simulink model "esp32_digital_output_demo"  (R2022a)
settings: Solver=FixedStepDiscrete  StartTime=0.0  StopTime=inf  RelTol=1e-3  EnableMultiTasking=on
undefined symbols (not defined in the file): ESP, IDF
libraries: simulink x9, esp32_io_lib x1, esp32_device_config_lib x1
settings Model: Creator=rnd1  LastModifiedBy=62-603
settings SolverCC: AlgebraicLoopSolver=TrustRegion  PositivePriorityOrder=on  AutoInsertRateTranBlk=on
settings DataIOCC: ReturnWorkspaceOutputs=off
settings OptimizationCC: DefaultParameterBehavior=Inlined  EnhancedBackFolding=on  PassReuseOutputArgsAs=Individual arguments  OptimizeBlockOrder=speed  DifferentSizesBufferReuse=on  OptimizationCustomize=off  EfficientTunableParamExpr=on
settings DebuggingCC: ParameterTunabilityLossMsg=error  UnconnectedInputMsg=warning  UnconnectedOutputMsg=warning  UnconnectedLineMsg=warning  SFMachineParentedDataDiag=warning  ArithmeticOperatorsInVariantConditions=warning
settings HardwareCC: ProdBitPerPointer=32  ProdBitPerSizeT=32  ProdBitPerPtrDiffT=32  ProdLargestAtomicFloat=None  ProdIntDivRoundTo=Undefined  ProdEndianess=Unspecified  ProdWordSize=32  ProdHWDeviceType=Cadence Design Systems (Tensilica)->Xtensa® single-/dual-core 32-bit LX6 microprocessor
settings SFSimCC: MATLABDynamicMemAlloc=off  CustomCodeUndefinedFunction=UseInterfaceOnly
settings RTWCC: Description=Waijung 2 ESP32 target  SystemTargetFile=esp32.tlc  GenCodeOnly=on  MakeCommand=make_rtw TMF=1  GenerateMakefile=off  TemplateMakefile=ert_default_tmf  GenerateReport=on  RetainRTWFile=on  IncludeHyperlinkInReport=on  LaunchReport=on  GenerateTraceInfo=on  GenerateTraceReport=on  GenerateTraceReportSl=on  GenerateTraceReportSf=on  GenerateTraceReportEml=on
settings CodeAppCC: ForceParamTrailComments=on  IgnoreCustomStorageClasses=off  OperatorAnnotations=on  SimulinkDataObjDesc=on  SFDataObjDesc=on  InsertBlockDesc=on
settings ERTTargetCC: TargetLangStandard=C99 (ISO)  UseToolchainInfoCompliant=off  InlinedParameterPlacement=NonHierarchical  ERTSrcFileBannerTemplate=esp32_code_template.cgt  ERTHdrFileBannerTemplate=esp32_code_template.cgt  ERTDataSrcFileTemplate=esp32_code_template.cgt  ERTDataHdrFileTemplate=esp32_code_template.cgt  ERTCustomFileTemplate=esp32_file_process.tlc

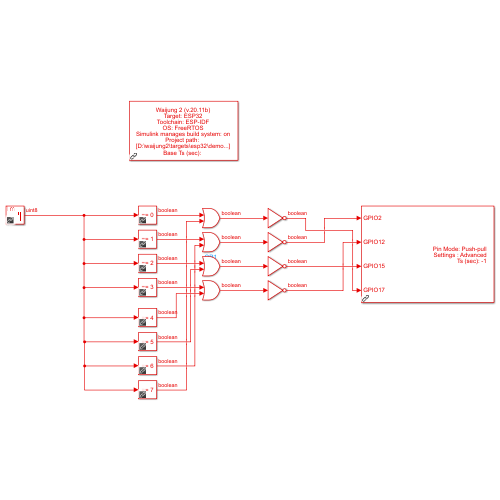
[thumbnail: Simulink's stored preview of the top-level diagram]
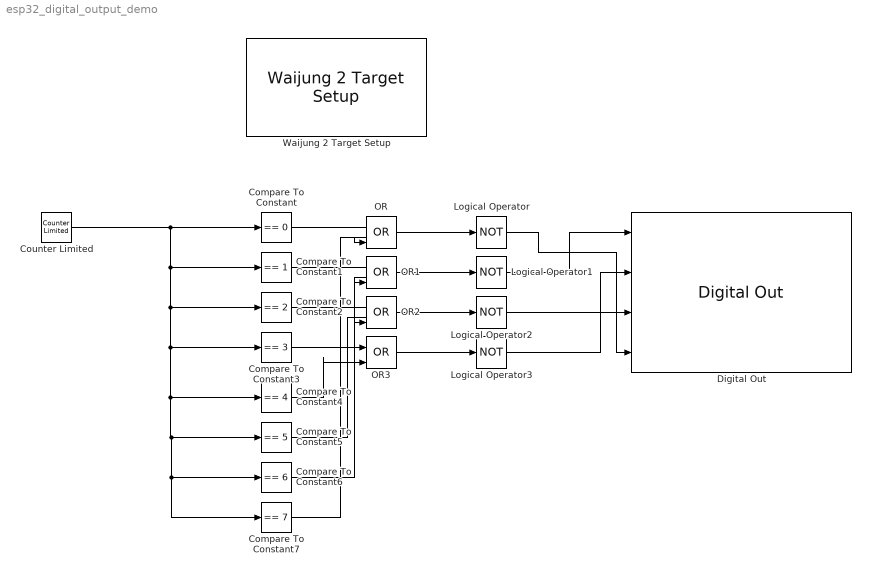
== system esp32_digital_output_demo ==
  Compare To Constant : simulink/Logic and Bit Operations/Compare To Constant  relop===  const=0  OutDataTypeStr=boolean
  Compare To Constant1 : simulink/Logic and Bit Operations/Compare To Constant  relop===  const=1  OutDataTypeStr=boolean
  Compare To Constant2 : simulink/Logic and Bit Operations/Compare To Constant  relop===  const=2  OutDataTypeStr=boolean
  Compare To Constant3 : simulink/Logic and Bit Operations/Compare To Constant  relop===  const=3  OutDataTypeStr=boolean
  Compare To Constant4 : simulink/Logic and Bit Operations/Compare To Constant  relop===  const=4  OutDataTypeStr=boolean
  Compare To Constant5 : simulink/Logic and Bit Operations/Compare To Constant  relop===  const=5  OutDataTypeStr=boolean
  Compare To Constant6 : simulink/Logic and Bit Operations/Compare To Constant  relop===  const=6  OutDataTypeStr=boolean
  Compare To Constant7 : simulink/Logic and Bit Operations/Compare To Constant  relop===  const=7  OutDataTypeStr=boolean
  Counter Limited : simulink/Sources/Counter Limited  uplimit=7  tsamp=0.3
  Digital Out : esp32_io_lib/Digital Out  blockid=DigitalOut  settings=Advanced  pin0=off  pin1=off  pin2=on  pin3=off  pin4=off  pin5=off  pin6=off  pin7=off  pin8=off  pin9=off  pin10=off  pin11=off  pin12=on  pin13=off  pin14=off  pin15=on  pin16=off  pin17=on  pin18=off  pin19=off  pin20=off  pin21=off  pin22=off  pin23=off  pin24=off  pin25=off  pin26=off  pin27=off  pin28=off  pin29=off  pin30=off  pin31=off  pin32=off  pin33=off  pin34=off  pin35=off  pin36=off  pin37=off  pin38=off  pin39=off  pin40=off  pin41=off  pin42=off  pin43=off  pin44=off  pin45=off  pin_initialize=on  pin_mode=Push-pull  sampletime=-1  drive_capability=Normal (default)  pin_hold=Disable  deep_sleep_pin_hold=Disable  pin_array="[0  0  1  0  0  0  0  0  0  0  0  0  1  0  0  1  0  1  0  0  0  0  0  0  0  0  0  0  0  0  0  0  0  0  0  0  0  0  0  0  0  0  0  0  0  0]"  inport_num=4  drive_capability_define=GPIO_DRIVE_CAP_2  pin_hold_define=off  pin_mode_define=GPIO_MODE_OUTPUT  deep_sleep_pin_hold_define=off  pin_string=((1ULL<<2) | (1ULL<<12) | (1ULL<<15) | (1ULL<<17))
      settings: SourceProductName=Waijung 2 Blockset
  Logical Operator{,1..3} (4 alike) : Logic  Operator=NOT  IconShape=distinctive  AllPortsSameDT=off  OutDataTypeStr=boolean
  OR{,1..3} (4 alike) : Logic  Operator=OR  IconShape=distinctive  AllPortsSameDT=off  OutDataTypeStr=boolean
  Waijung 2 Target Setup : esp32_device_config_lib/Waijung 2 Target Setup  toolchain=ESP-IDF  os=FreeRTOS  sampletime=-1  simulink_managebuildsystem=on  projectpath=D:\waijung2\targets\esp32\demo\digital_output_demo\esp32_digital_output_demo_esp32_build_system  espidfpath=C:\msys32\home\skris\esp\esp-idf  auto_compile_download=on  blockid=Waijung2TargetSetup  target=ESP32  waijungversion=20.11b  defaultstacksize=2048  basepriority=0  highestpriority=16  generate_baserate_task=on  esp32flashsize=4MB  esp32comport=COM3
      settings: SourceProductName=Waijung 2 Blockset
  wires:
  Counter Limited/1 -> Compare To Constant1/1, Compare To Constant2/1, Compare To Constant7/1, Compare To Constant6/1, Compare To Constant5/1, Compare To Constant4/1, Compare To Constant3/1, Compare To Constant/1
  Compare To Constant/1 -> OR/1
  Compare To Constant7/1 -> OR/2
  Compare To Constant1/1 -> OR1/1
  Compare To Constant6/1 -> OR1/2
  Compare To Constant2/1 -> OR2/1
  Compare To Constant5/1 -> OR2/2
  Compare To Constant3/1 -> OR3/1
  Compare To Constant4/1 -> OR3/2
  OR/1 -> Logical Operator/1
  OR1/1 -> Logical Operator1/1
  OR2/1 -> Logical Operator2/1
  OR3/1 -> Logical Operator3/1
  Logical Operator/1 -> Digital Out/4
  Logical Operator3/1 -> Digital Out/2
  Logical Operator2/1 -> Digital Out/3
  Logical Operator1/1 -> Digital Out/1
